simulink model "simulink_ejercicio3"  (R2023a)
settings: Solver=VariableStepAuto  StartTime=0.0  StopTime=10.0  RelTol=1e-3
values from neighbouring files (symbols this model uses):
  b1 = 1000    [mov_traslacional.m]    (also in parametros_ejercicio3.m)
  k1 = 16182    [mov_traslacional.m]    (also in parametros_ejercicio3.m)
  k2 = 19000    [mov_traslacional.m]    (also in parametros_ejercicio3.m)
  m1 = 290    [mov_traslacional.m]    (also in parametros_ejercicio3.m)
  m2 = 59    [mov_traslacional.m]    (also in parametros_ejercicio3.m)
settings Model: Creator=penqu  LastModifiedBy=penqu

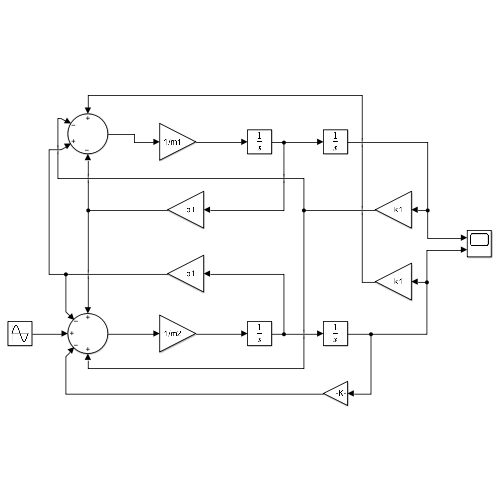
[thumbnail: Simulink's stored preview of the top-level diagram]
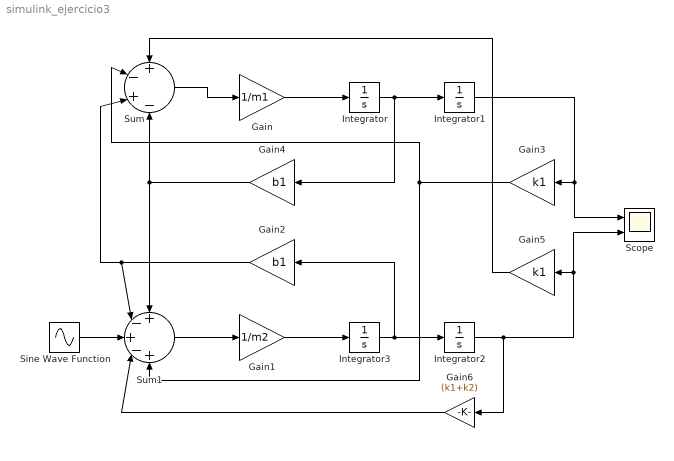
== system simulink_ejercicio3 ==
  Gain : Gain  Gain=1/m1
  Gain1 : Gain  Gain=1/m2
  Gain2 : Gain  Gain=b1
  Gain3 : Gain  Gain=k1
  Gain4 : Gain  Gain=b1
  Gain5 : Gain  Gain=k1
  Gain6 : Gain  Gain=(k1+k2)
  Integrator{,1..3} (4 alike) : Integrator
  Scope : Scope  NumInputPorts=2
  Sine Wave Function : Sin  Amplitude=0.05*k2  Frequency=0.5*pi  SampleTime=0
  Sum : Sum  Inputs=+-+-
  Sum1 : Sum  Inputs=+-+-+
  wires:
  Sum1/1 -> Gain1/1
  Integrator3/1 -> Gain2/1, Integrator2/1
  Gain1/1 -> Integrator3/1
  Integrator/1 -> Gain4/1, Integrator1/1
  Integrator1/1 -> Scope/1, Gain3/1
  Integrator2/1 -> Gain6/1, Scope/2, Gain5/1
  Sum/1 -> Gain/1
  Gain/1 -> Integrator/1
  Gain4/1 -> Sum1/1, Sum/4
  Gain2/1 -> Sum/3, Sum1/2
  Gain3/1 -> Sum/2, Sum1/5
  Gain6/1 -> Sum1/4
  Gain5/1 -> Sum/1
  Sine Wave Function/1 -> Sum1/3
